simulink model "Modell_13_3"  (R2018a)
settings: Solver=VariableStepAuto  StartTime=0.0  StopTime=10.0  RelTol=1e-3
settings Model: Creator=Uni  LastModifiedBy=Uni

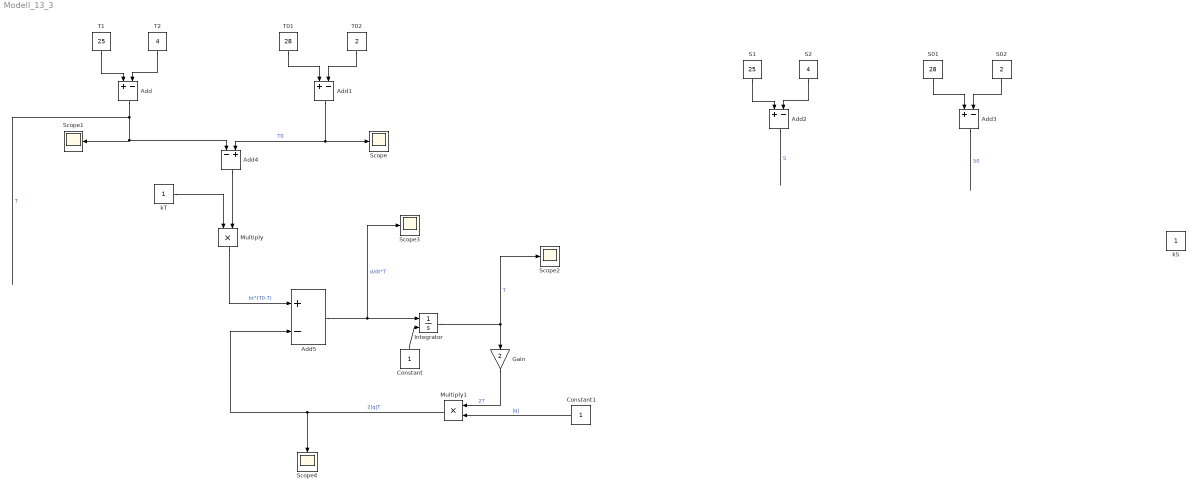
== system Modell_13_3 ==
  Add{,1..3,5} (5 alike) : Sum  Inputs=+-
  Add4 : Sum  Inputs=-+
  Constant : Constant
  Constant1 : Constant
  Gain : Gain  Gain=2
  Integrator : Integrator  InitialConditionSource=external
  Multiply : Product
  Multiply1 : Product
  S01 : Constant  Value=28
  S02 : Constant  Value=2
  S1 : Constant  Value=25
  S2 : Constant  Value=4
  Scope{,1..4} (5 alike) : Scope
  T01 : Constant  Value=28
  T02 : Constant  Value=2
  T1 : Constant  Value=25
  T2 : Constant  Value=4
  kS : Constant
  kT : Constant
  wires:
  T1/1 -> Add/1
  T2/1 -> Add/2
  Add/1 -> Scope1/1, Add4/1  "T"
  T01/1 -> Add1/1
  T02/1 -> Add1/2
  Add1/1 -> Add4/2, Scope/1  "T0"
  Add3/1 -> ?  "S0"
  S02/1 -> Add3/2
  S01/1 -> Add3/1
  Add2/1 -> ?  "S"
  S2/1 -> Add2/2
  S1/1 -> Add2/1
  Add4/1 -> Multiply/2
  kT/1 -> Multiply/1
  Multiply/1 -> Add5/1  "kt*(T0-T)"
  Constant/1 -> Integrator/2
  Add5/1 -> Scope3/1, Integrator/1  "d/dt*T"
  Integrator/1 -> Gain/1, Scope2/1  "T"
  Gain/1 -> Multiply1/1  "2T"
  Multiply1/1 -> Add5/2, Scope4/1  "2|q|T"
  Constant1/1 -> Multiply1/2  "|q|"
